simulink model "Caso9ControleRele"  (R2015a)
settings: Solver=ode45  StartTime=0.0  StopTime=0.5
libraries: simulink x6
settings Model: Creator=user  LastModifiedBy=user
settings SolverCC: ShapePreserveControl=EnableAll  ZeroCrossControl=DisableAll

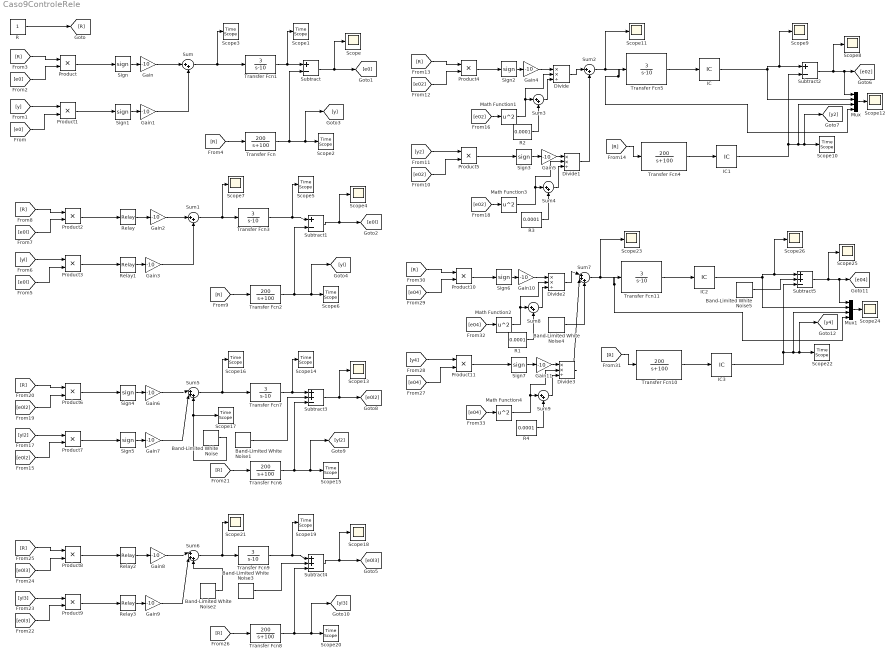
== system Caso9ControleRele ==
  Band-Limited White Noise{,2..5} (5 alike) : simulink/Sources/Band-Limited White Noise  Cov=[0.00001]  Ts=0.001  seed=[23341]
  Band-Limited White Noise1 : simulink/Sources/Band-Limited White Noise  Cov=[0.00001]  Ts=0.001  seed=[23347]
  Divide{,1..3} (4 alike) : Product  Inputs=**/
  Gain{,1..11} (12 alike) : Gain  Gain=-10
  IC : InitialCondition  Value=6
  IC1 : InitialCondition  Value=0
  IC2 : InitialCondition  Value=6
  IC3 : InitialCondition  Value=0
  Math Function{1..4} (4 alike) : Math  Operator=square  SaturateOnIntegerOverflow=on
  Mux : Mux
  Mux1 : Mux
  Product{,1..11} (12 alike) : Product
  R : Constant
  R{1..4} (4 alike) : Constant  Value=0.0001
  Relay{,1..3} (4 alike) : Relay  OnSwitchValue=0.05  OffSwitchValue=-0.05  OffOutputValue=-1
  Scope{,4,7..9,11..13,18,21,23..26} (14 alike) : Scope
      Scope settings: YMin=-1.73472e-18  YMax=0.02
      Scope11 settings: TimeRange=10  YMin=-7  YMax=-0.5
      Scope12 settings: YMin=-7  SaveName=ScopeData3
      Scope13 settings: YMin=-1.73472e-18  YMax=0.02  SaveName=ScopeData4
      Scope18 settings: YMin=-1.73472e-18  YMax=0.02  SaveName=ScopeData12
      Scope21 settings: YMin=-525  YMax=-475  SaveName=ScopeData15
      Scope23 settings: TimeRange=10  YMin=-7  YMax=-0.5  SaveName=ScopeData17
      Scope24 settings: YMin=-7  SaveName=ScopeData18
      Scope25 settings: YMin=0.002  YMax=0.0028  SaveName=ScopeData19
      Scope26 settings: TimeRange=10  YMin=2.00681  YMax=2.007  SaveName=ScopeData20
      Scope4 settings: YMin=-1.73472e-18  YMax=0.02  SaveName=ScopeData2
      Scope7 settings: YMin=-525  YMax=-475  SaveName=ScopeData6
      Scope8 settings: YMin=0.002  YMax=0.0028  SaveName=ScopeData8
      Scope9 settings: TimeRange=10  YMin=2.00681  YMax=2.007  SaveName=ScopeData9
  Scope{1..3,5..6,10,14..17,19..20,22} (13 alike) : TimeScope
  Sign{,1..7} (8 alike) : Signum
  Subtract : Sum  Inputs=+-
  Subtract1 : Sum  Inputs=+-
  Subtract2 : Sum  Inputs=+-
  Subtract3 : Sum  Inputs=++-
  Subtract4 : Sum  Inputs=++-
  Subtract5 : Sum  Inputs=++-
  Sum{,1..4,8..9} (7 alike) : Sum  Inputs=|++
  Sum5 : Sum  Inputs=|+++
  Sum6 : Sum  Inputs=|+++
  Sum7 : Sum  Inputs=|+++
  Transfer Fcn{,2,4,6,8,10} (6 alike) : TransferFcn  Numerator=[200]  Denominator=[1 100]
  Transfer Fcn{1,3,5,7,9,11} (6 alike) : TransferFcn  Numerator=[3]  Denominator=[1 -10]
  wires:
  Sum/1 -> Scope3/1, Transfer Fcn1/1
  Sign/1 -> Gain/1
  Sign1/1 -> Gain1/1
  Gain1/1 -> Sum/2
  Gain/1 -> Sum/1
  Product/1 -> Sign/1
  Product1/1 -> Sign1/1
  [e0] -> Product1/2
  [y] -> Product1/1
  [e0] -> Product/2
  [R] -> Product/1
  [R] -> Transfer Fcn/1
  Transfer Fcn1/1 -> Scope1/1, Subtract/1
  Transfer Fcn/1 -> Subtract/2, [y], Scope2/1
  Subtract/1 -> Scope/1, [e0]
  R/1 -> [R]
  Sum1/1 -> Scope7/1, Transfer Fcn3/1
  Relay/1 -> Gain2/1
  Relay1/1 -> Gain3/1
  Gain3/1 -> Sum1/2
  Gain2/1 -> Sum1/1
  Product2/1 -> Relay/1
  Product3/1 -> Relay1/1
  [e0l] -> Product3/2
  [yl] -> Product3/1
  [e0l] -> Product2/2
  [R] -> Product2/1
  [R] -> Transfer Fcn2/1
  Transfer Fcn3/1 -> Scope5/1, Subtract1/1
  Transfer Fcn2/1 -> Subtract1/2, [yl], Scope6/1
  Subtract1/1 -> Scope4/1, [e0l]
  Sum2/1 -> Scope11/1, Transfer Fcn5/1, Mux/4
  Sign2/1 -> Gain4/1
  Sign3/1 -> Gain5/1
  Product4/1 -> Sign2/1
  Product5/1 -> Sign3/1
  [e02] -> Product5/2
  [y2] -> Product5/1
  [e02] -> Product4/2
  [R] -> Product4/1
  [R] -> Transfer Fcn4/1
  Transfer Fcn4/1 -> IC1/1
  Subtract2/1 -> Scope8/1, Mux/1, [e02]
  Sum3/1 -> Divide/3
  Gain4/1 -> Divide/1
  Divide/1 -> Sum2/1
  [e02] -> Math Function1/1
  R2/1 -> Sum3/2
  Sum4/1 -> Divide1/3
  [e02] -> Math Function3/1
  R3/1 -> Sum4/2
  Divide1/1 -> Sum2/2
  Math Function1/1 -> Divide/2, Sum3/1
  Math Function3/1 -> Divide1/2, Sum4/1
  Gain5/1 -> Divide1/1
  Mux/1 -> Scope12/1
  Transfer Fcn5/1 -> IC/1
  IC/1 -> Scope9/1, Subtract2/1, Mux/2
  IC1/1 -> Subtract2/2, Mux/3, [y2], Scope10/1
  Sum5/1 -> Scope16/1, Transfer Fcn7/1
  Sign4/1 -> Gain6/1
  Sign5/1 -> Gain7/1
  Gain7/1 -> Sum5/2
  Gain6/1 -> Sum5/1
  Product6/1 -> Sign4/1
  Product7/1 -> Sign5/1
  [e0l2] -> Product7/2
  [yl2] -> Product7/1
  [e0l2] -> Product6/2
  [R] -> Product6/1
  [R] -> Transfer Fcn6/1
  Transfer Fcn7/1 -> Scope14/1, Subtract3/1
  Transfer Fcn6/1 -> Subtract3/3, [yl2], Scope15/1
  Subtract3/1 -> Scope13/1, [e0l2]
  Band-Limited White Noise1/1 -> Subtract3/2
  Band-Limited White Noise/1 -> Scope17/1, Sum5/3
  Sum6/1 -> Scope21/1, Transfer Fcn9/1
  Relay2/1 -> Gain8/1
  Relay3/1 -> Gain9/1
  Gain9/1 -> Sum6/2
  Gain8/1 -> Sum6/1
  Product8/1 -> Relay2/1
  Product9/1 -> Relay3/1
  [e0l3] -> Product9/2
  [yl3] -> Product9/1
  [e0l3] -> Product8/2
  [R] -> Product8/1
  [R] -> Transfer Fcn8/1
  Transfer Fcn9/1 -> Scope19/1, Subtract4/1
  Transfer Fcn8/1 -> Subtract4/3, [yl3], Scope20/1
  Subtract4/1 -> Scope18/1, [e0l3]
  Band-Limited White Noise3/1 -> Subtract4/2
  Band-Limited White Noise2/1 -> Sum6/3
  Sum7/1 -> Scope23/1, Transfer Fcn11/1, Mux1/4
  Sign6/1 -> Gain10/1
  Sign7/1 -> Gain11/1
  Product10/1 -> Sign6/1
  Product11/1 -> Sign7/1
  [e04] -> Product11/2
  [y4] -> Product11/1
  [e04] -> Product10/2
  [R] -> Product10/1
  [R] -> Transfer Fcn10/1
  Transfer Fcn10/1 -> IC3/1
  Subtract5/1 -> Scope25/1, Mux1/1, [e04]
  Sum8/1 -> Divide2/3
  Gain10/1 -> Divide2/1
  Divide2/1 -> Sum7/1
  [e04] -> Math Function2/1
  R1/1 -> Sum8/2
  Sum9/1 -> Divide3/3
  [e04] -> Math Function4/1
  R4/1 -> Sum9/2
  Divide3/1 -> Sum7/2
  Math Function2/1 -> Divide2/2, Sum8/1
  Math Function4/1 -> Divide3/2, Sum9/1
  Gain11/1 -> Divide3/1
  Mux1/1 -> Scope24/1
  Transfer Fcn11/1 -> IC2/1
  IC2/1 -> Scope26/1, Subtract5/1, Mux1/2
  IC3/1 -> Subtract5/3, Mux1/3, [y4], Scope22/1
  Band-Limited White Noise5/1 -> Subtract5/2
  Band-Limited White Noise4/1 -> Sum7/3
